simulink model "simulator"  (R2020b)
settings: Solver=ode3  StartTime=0.0  StopTime=5000  FixedStep=1  RelTol=1e-3
InitFcn:
  | clear all
  | clc
  | 
  | %run config_Houston.m
  | run config_Malaga.m
  | 
  | load('PBNsim_buses');
StartFcn:
  | rng('shuffle');
values from neighbouring files (symbols this model uses):
  WP = zeros(numWP,3)    [config_Malaga.m]
  WPabort = 9    [config_Malaga.m]
  WPnext = [   2 ... (first row only)    [config_Malaga.m]
  WPspeed = [ 240 ... (first row only)    [config_Malaga.m]
undefined symbols (not defined in the file or in its folder): m, n
libraries: AC x24
(part 1 of 2)
settings Model: OrderedModelArguments=off  Creator=rcasado  LastModifiedBy=usuario
settings DataIOCC: ReturnWorkspaceOutputs=off
settings DebuggingCC: ArithmeticOperatorsInVariantConditions=warning
settings SFSimCC: SimUseLocalCustomCode=off  CustomCodeUndefinedFunction=UseInterfaceOnly
settings RTWCC: RTWUseLocalCustomCode=off
settings CodeAppCC: StateflowObjectComments=on

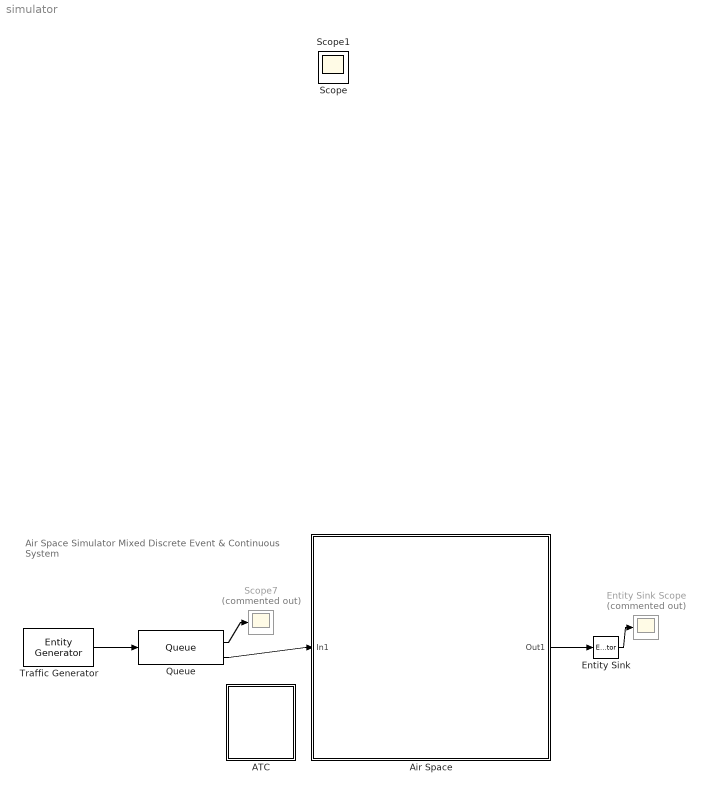
== system simulator ==
  note: Air Space Simulator
      | Mixed Discrete Event & Continuous System
  ATC : Subsystem
      mask Display: image('assets/ATC.svg');
  Air Space : Subsystem
  Entity Sink : EntityTerminator  InputPortMessageModes=m  EntryAction=|  NumberEntitiesArrived=on
      | coder.extrinsic('get_param')
      | currentTime = 0;
      | %currentTime = get_param('simulator18b','SimulationTime');
      | currentTime = get_param(get_param(0,'CurrentSystem'),'SimulationTime');
      | flightTime  = currentTime -entity.startTime;
      | 
      | fprintf('%5.0f: aeronave %3.0f aterriza en %4.0f s\n',...
      |     currentTime,...
      |     entity.flightId,...
      |     flightTime);
      settings: OutputPortMap=o0
  Entity Sink Scope : Scope  Commented=on
  Queue : Queue  InputPortMessageModes=m  OutputPortMessageModes=n,m  Capacity=10  PrioritySource=PriorityAttributeName  BlockedAction=|  NumberEntitiesInBlock=on
      | coder.extrinsic('set_param','gcs');
      | set_param(gcs, 'SimulationCommand', 'stop');
      | 
      | disp('Simulación interrumpida: no hay aviones suficientes para satisfacer la demanda de tráfico aéreo');
      settings: OutputPortMap=o1,o5
  Scope7 : Scope  Commented=on
  Traffic Generator : EntityGenerator  OutputPortMessageModes=m  TimeSource=MATLAB action  Period=120  IntergenerationTimeAction=|  GenerateAction=|  AttributeName=flightId|startTime  AttributeInitialValue=0|0  EntityType=Structured  EntityTypeName=aircraft
      IntergenerationTimeAction=|
      | % Pattern: Repeating Sequence
      | persistent SEQ1;
      | persistent idx1;
      | if isempty(SEQ1)
      |     
      |     % PRUEBAS EN MALAGA: 
      |     SEQ1 = [ 90 90 90 90 90 90 90 90 90 90 90         200        90 ];
      |     
      |     idx1 = 1;
      | end
      | 
      | dt = SEQ1(idx1);
      | 
      | if idx1 == numel(SEQ1)
      |     idx1 = 1;    
      | else
      |     idx1 = idx1 + 1;
      | end
      | 
      | %% para generar un solo avion descomentar lo siguiente
      | % dt = inf
      GenerateAction=|
      | persistent next_flightId;
      | if isempty(next_flightId)
      |     next_flightId = 1;
      | end
      | entity.flightId = next_flightId;
      | next_flightId = next_flightId + 1;
      | 
      | coder.extrinsic('get_param')
      | %entity.startTime = get_param('simulator18b','SimulationTime');
      | entity.startTime = get_param(get_param(0,'CurrentSystem'),'SimulationTime');
      | fprintf('%5.0f: aeronave %3.0f entra en espacio aereo\n',entity.startTime,entity.flightId);
  Scope : Scope
  Scope1 : Scope
  wires:
  Traffic Generator/1 -> Queue/1
  Queue/1 -> Scope7/1
  Entity Sink/1 -> Entity Sink Scope/1
  Queue/2 -> Air Space/1(In1)
  Air Space/1(Out1) -> Entity Sink/1

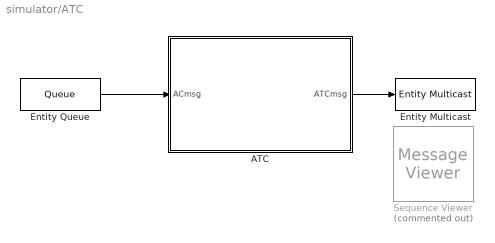
== system simulator/ATC ==
  ATC : Stateflow chart  TreatAsAtomicUnit=on
  Entity Multicast : EntityMulticast  InputPortMessageModes=m  MulticastTag=ATCcomm
  Entity Queue : Queue  OutputPortMessageModes=m  Capacity=100  EntityArrivalSource=Multicast  MulticastTag=ACcomm
  Sequence Viewer : MessageViewer  Commented=on  History=1000
  wires:
  ATC/1(ATCmsg) -> Entity Multicast/1
  Entity Queue/1 -> ATC/1(ACmsg)

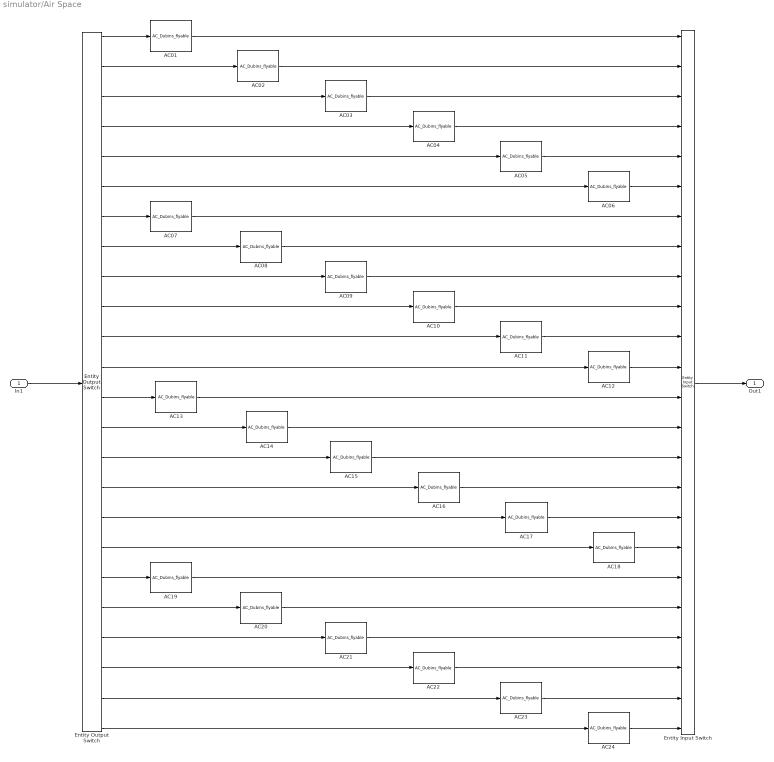
== system simulator/Air Space ==
  In1 : Inport
  AC01 : AC/AC_Dubins_flyable  SystemSampleTime=-1  VariantActivationTime=update diagram  Latency=0  AutoFrameSizeCalculation=off
  AC02 : AC/AC_Dubins_flyable  SystemSampleTime=-1  VariantActivationTime=update diagram  Latency=0  AutoFrameSizeCalculation=off
  AC03 : AC/AC_Dubins_flyable  SystemSampleTime=-1  VariantActivationTime=update diagram  Latency=0  AutoFrameSizeCalculation=off
  AC04 : AC/AC_Dubins_flyable  SystemSampleTime=-1  VariantActivationTime=update diagram  Latency=0  AutoFrameSizeCalculation=off
  AC05 : AC/AC_Dubins_flyable  SystemSampleTime=-1  VariantActivationTime=update diagram  Latency=0  AutoFrameSizeCalculation=off
  AC06 : AC/AC_Dubins_flyable  SystemSampleTime=-1  VariantActivationTime=update diagram  Latency=0  AutoFrameSizeCalculation=off
  AC07 : AC/AC_Dubins_flyable  SystemSampleTime=-1  VariantActivationTime=update diagram  Latency=0  AutoFrameSizeCalculation=off
  AC08 : AC/AC_Dubins_flyable  SystemSampleTime=-1  VariantActivationTime=update diagram  Latency=0  AutoFrameSizeCalculation=off
  AC09 : AC/AC_Dubins_flyable  SystemSampleTime=-1  VariantActivationTime=update diagram  Latency=0  AutoFrameSizeCalculation=off
  AC{10..24} (15 alike) : AC/AC_Dubins_flyable  SystemSampleTime=-1  VariantActivationTime=update diagram  Latency=0  AutoFrameSizeCalculation=off
  Entity Input Switch : EntityInputSwitch  InputPortMessageModes=m,m,m,m,m,m,m,m,m,m,m,m,m,m,m,m,m,m,m,m,m,m,m,m  OutputPortMessageModes=m  NumberInputPorts=24
      settings: InputPortMap=u1,u2,u3,u4,u5,u6,u7,u8,u9,u10,u11,u12,u13,u14,u15,u16,u17,u18,u19,u20,u21,u22,u23,u24
  Entity Output Switch : EntityOutputSwitch  InputPortMessageModes=m  OutputPortMessageModes=m,m,m,m,m,m,m,m,m,m,m,m,m,m,m,m,m,m,m,m,m,m,m,m  NumberOutputPorts=24  SwitchAttributeName=Attribute1
      settings: OutputPortMap=o0,o1,o2,o3,o4,o5,o6,o7,o8,o9,o10,o11,o12,o13,o14,o15,o16,o17,o18,o19,o20,o21,o22,o23
  Out1 : Outport
  wires:
  Entity Output Switch/1 -> AC01/1
  Entity Output Switch/3 -> AC03/1
  Entity Output Switch/4 -> AC04/1
  AC04/1 -> Entity Input Switch/4
  AC02/1 -> Entity Input Switch/2
  AC01/1 -> Entity Input Switch/1
  AC03/1 -> Entity Input Switch/3
  In1/1 -> Entity Output Switch/1
  Entity Input Switch/1 -> Out1/1
  Entity Output Switch/2 -> AC02/1
  Entity Output Switch/5 -> AC05/1
  Entity Output Switch/6 -> AC06/1
  Entity Output Switch/8 -> AC08/1
  AC09/1 -> Entity Input Switch/9
  AC07/1 -> Entity Input Switch/7
  Entity Output Switch/9 -> AC09/1
  Entity Output Switch/11 -> AC11/1
  AC10/1 -> Entity Input Switch/10
  Entity Output Switch/12 -> AC12/1
  Entity Output Switch/10 -> AC10/1
  Entity Output Switch/20 -> AC20/1
  AC21/1 -> Entity Input Switch/21
  AC19/1 -> Entity Input Switch/19
  Entity Output Switch/21 -> AC21/1
  Entity Output Switch/23 -> AC23/1
  AC22/1 -> Entity Input Switch/22
  Entity Output Switch/24 -> AC24/1
  Entity Output Switch/22 -> AC22/1
  AC05/1 -> Entity Input Switch/5
  AC06/1 -> Entity Input Switch/6
  Entity Output Switch/19 -> AC19/1
  AC24/1 -> Entity Input Switch/24
  AC23/1 -> Entity Input Switch/23
  Entity Output Switch/13 -> AC13/1
  Entity Output Switch/14 -> AC14/1
  Entity Output Switch/15 -> AC15/1
  Entity Output Switch/16 -> AC16/1
  Entity Output Switch/17 -> AC17/1
  Entity Output Switch/18 -> AC18/1
  AC18/1 -> Entity Input Switch/18
  AC17/1 -> Entity Input Switch/17
  AC16/1 -> Entity Input Switch/16
  AC15/1 -> Entity Input Switch/15
  AC13/1 -> Entity Input Switch/13
  AC12/1 -> Entity Input Switch/12
  AC11/1 -> Entity Input Switch/11
  Entity Output Switch/7 -> AC07/1
  AC08/1 -> Entity Input Switch/8
  AC14/1 -> Entity Input Switch/14
  AC20/1 -> Entity Input Switch/20
